simulink model "Mission_Server_QBot2e_IO_Check_r2018a"  (Simulink 9.1)
settings: Solver=ode2  StartTime=0.0  StopTime=inf  FixedStep=0.001  RelTol=1e-3  EnableMultiTasking=on
undefined symbols (not defined in the file): Host
libraries: quarc_library x13, simulink x4
settings Model: Creator=Admin  LastModifiedBy=user  SimulationMode=external  ExtModeTrigDuration=10000
settings SolverCC: PositivePriorityOrder=on
settings DataIOCC: SaveFormat=Dataset
settings OptimizationCC: LifeSpan=auto
settings DebuggingCC: UnderspecifiedInitializationDetection=Simplified  MergeDetectMultiDrivingBlocksExec=error
settings HardwareCC: ProdBitPerPointer=64  ProdBitPerSizeT=64  ProdBitPerPtrDiffT=64  ProdLargestAtomicFloat=Float  ProdIntDivRoundTo=Zero  ProdEndianess=LittleEndian  ProdWordSize=64  ProdHWDeviceType=Intel->x86-64 (Windows64)
settings ModelReferenceCC: PropagateSignalLabelsOutOfModel=on
settings RTWCC: Description=QUARC Win64 Target Using Toolchain  SystemTargetFile=quarc_win64.tlc  TemplateMakefile=quarc_default_tmf  Toolchain=QUARC win64 | nmake (64-bit Windows)  BuildConfiguration=Faster Runs
settings STFCustomTargetCC: ConcurrentExecutionCompliant=on  UseToolchainInfoCompliant=on  SystemTargetFile=quarc_win64.tlc
settings GRTTargetCC: ParMdlRefBuildCompliant=off  CompOptLevelCompliant=off  MatFileLogging=off  CPPClassGenCompliant=off  ExtMode=on  ExtModeMexFile=quarc_comm  ExtModeMexArgs='-w -d %d -uri %u -d_IP_q tcpip://localhost:18000'

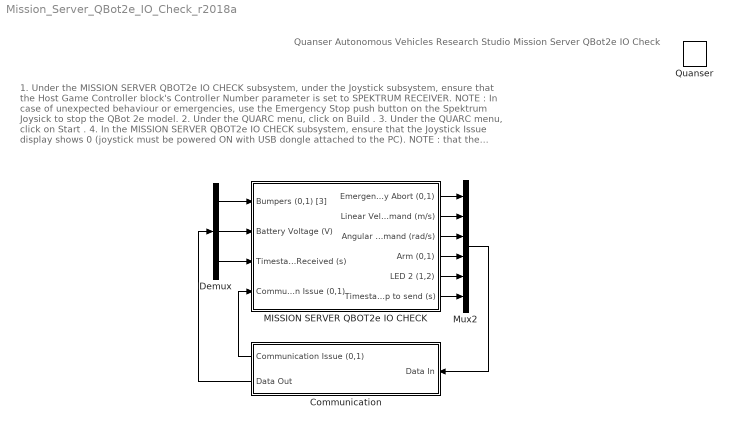
== system Mission_Server_QBot2e_IO_Check_r2018a ==
  note: 1. Under the MISSION SERVER QBOT2e IO CHECK subsystem, under the Joystick subsystem, ensure that the Host Game Controller block's Controller Number parameter is set to SPEKTRUM RECEIVER.
      | NOTE : In case of unexpected behaviour or emergencies, use the Emergency Stop push button on the Spektrum Joysick to stop the QBot 2e model.
      | 2. Under the QUARC menu, click on Build .
      | 3. Under the QUARC menu, click on Start .
      | 4. In the MISSION SERVER QBOT2e IO CHECK subsystem, ensure that the Joystick Issue display shows 0 (joystick must be powered ON with USB dongle attached to the PC).
      | NOTE : that the Loop-back Time (s) display SHOULD display an increasing time value until the QBot 2e Stabilizer model is running. When it is running, this display should oscillate around a small value (~0.004 to 0.005s).
  note: Quanser Autonomous Vehicles Research Studio
      | Mission Server QBot2e IO Check
  Communication : Subsystem
  Demux : Demux  Outputs=[3 1 1 ]
  MISSION SERVER QBOT2e IO CHECK : Subsystem
  Mux2 : Mux  Inputs=6
  Quanser : quarc_library/Logos/Quanser
  wires:
  Communication/2(Data Out) -> Demux/1
  Demux/3 -> MISSION SERVER QBOT2e IO CHECK/3(Timestamp Received (s))
  Demux/1 -> MISSION SERVER QBOT2e IO CHECK/1(Bumpers (0,1) [3])
  Demux/2 -> MISSION SERVER QBOT2e IO CHECK/2(Battery Voltage (V))
  Communication/1(Communication Issue (0,1)) -> MISSION SERVER QBOT2e IO CHECK/4(Communication Issue (0,1))
  MISSION SERVER QBOT2e IO CHECK/1(Emergency Abort (0,1)) -> Mux2/1
  MISSION SERVER QBOT2e IO CHECK/2(Linear Velocity Command (m/s)) -> Mux2/2
  MISSION SERVER QBOT2e IO CHECK/3(Angular Velocity Command (rad/s)) -> Mux2/3
  MISSION SERVER QBOT2e IO CHECK/4(Arm (0,1)) -> Mux2/4
  MISSION SERVER QBOT2e IO CHECK/5(LED 2 (1,2)) -> Mux2/5
  MISSION SERVER QBOT2e IO CHECK/6(Timestamp to send (s)) -> Mux2/6
  Mux2/1 -> Communication/1(Data In)

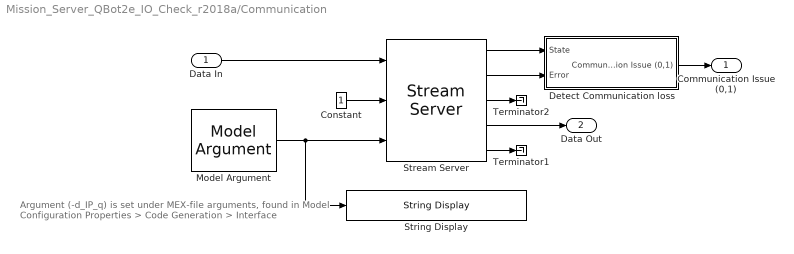
== system Mission_Server_QBot2e_IO_Check_r2018a/Communication ==
  note: Argument (-d_IP_q) is set under
      | MEX-file arguments, found in
      | Model Configuration Properties > Code Generation > Interface
  Data In : Inport
  Constant : Constant
  Detect Communication loss : Subsystem
  Model Argument : quarc_library/Sources/Signals/Model Argument  argument_name=d_IP_q  has_value=on  data_type_mode=Specify via dialog  data_type=char  max_length=80  default_value=0  variable_size=off
      settings: AttributesFormatString=(-%<argument_name>)  SourceProductName=QUARC Targets
  Stream Server : quarc_library/Communications/Basic/Stream Server  uri_source=External input port  uri=tcpip://localhost:18666  apply_uri_to_all_configs=off  send_buffer_size=1460  receive_buffer_size=1460  byte_order=little endian (Intel - LSB first)  optimization=Minimum latency  send_options=Send most recent data  receive_options=Receive most recent data  default_value=zeros(1,5)  sample_time=qc_get_step_size  active=off  implementation=Use blocking I/O in a separate thread  send_fifo_size=1  receive_fifo_size=1  send_priority=0  receive_priority=0  send_dimensions=off  receive_dimensions=off  max_dimensions=-1  data_type=double  type_expr=BusObject
  "String Display " : quarc_library/Strings/String Display  alignment=center  display_mode=Single line  sample_time=-1  use_new=off
      settings: SourceProductName=QUARC Targets
  Terminator1 : Terminator
  Terminator2 : Terminator
  Communication Issue (0,1) : Outport  VectorParamsAs1DForOutWhenUnconnected=off
  Data Out : Outport  Port=2  VectorParamsAs1DForOutWhenUnconnected=off
  wires:
  Stream Server/3 -> Terminator2/1
  Constant/1 -> Stream Server/2
  Stream Server/1 -> Detect Communication loss/1(State)
  Data In/1 -> Stream Server/1
  Model Argument/1 -> Stream Server/3, "String Display "/1
  Stream Server/4 -> Data Out/1
  Stream Server/5 -> Terminator1/1
  Stream Server/2 -> Detect Communication loss/2(Error)
  Detect Communication loss/1(Communication Issue (0,1)) -> Communication Issue (0,1)/1

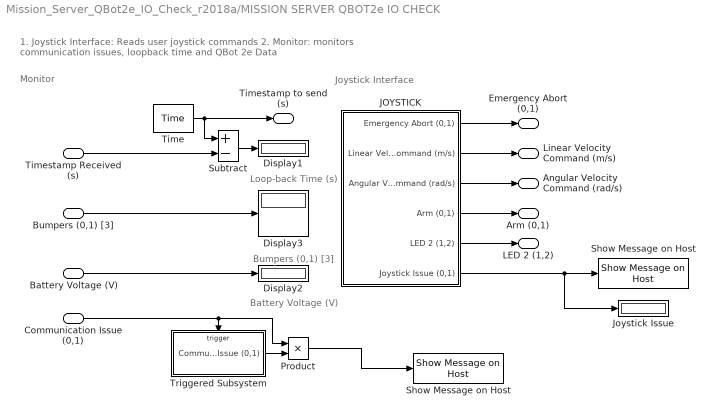
== system Mission_Server_QBot2e_IO_Check_r2018a/MISSION SERVER QBOT2e IO CHECK ==
  note: Monitor
  note: Joystick Interface
  note: 1. Joystick Interface: Reads user joystick commands
      | 2. Monitor: monitors communication issues, loopback time and QBot 2e Data
  note: Battery Voltage (V)
  note: Bumpers (0,1) [3]
  note: Loop-back Time (s)
  Bumpers (0,1) [3] : Inport
  Battery Voltage (V) : Inport  Port=2
  Timestamp Received (s) : Inport  Port=3
  Communication Issue (0,1) : Inport  Port=4
  Display1 : Display
  Display2 : Display
  Display3 : Display
  JOYSTICK : Subsystem
  Joystick Issue : Display
  Product : Product
  Show Message on Host : quarc_library/Sinks/Error Handling/Show Message on Host  message_type=Fixed error message  message_icon=Warning  message=Mission Server: Communication Issue with QBot2e
      settings: AttributesFormatString="\"%<message>\""  SourceProductName=QUARC Targets
  "Show Message on Host " : quarc_library/Sinks/Error Handling/Show Message on Host  message_type=Fixed error message  message_icon=Warning  message=Mission Server: Joystick Disconnected
      settings: AttributesFormatString="\"%<message>\""  SourceProductName=QUARC Targets
  Subtract : Sum  Inputs=+-
  Time : quarc_library/Sources/Time/Time  time_source=Wall clock  sample_time=qc_get_step_size
  Triggered Subsystem : Subsystem  TreatAsAtomicUnit=on
  Emergency Abort (0,1) : Outport  VectorParamsAs1DForOutWhenUnconnected=off
  Linear Velocity Command (m/s) : Outport  Port=2  VectorParamsAs1DForOutWhenUnconnected=off
  Angular Velocity Command (rad/s) : Outport  Port=3  VectorParamsAs1DForOutWhenUnconnected=off
  Arm (0,1) : Outport  Port=4  VectorParamsAs1DForOutWhenUnconnected=off
  LED 2 (1,2) : Outport  Port=5  VectorParamsAs1DForOutWhenUnconnected=off
  Timestamp to send (s) : Outport  Port=6  VectorParamsAs1DForOutWhenUnconnected=off
  wires:
  JOYSTICK/6(Joystick Issue (0,1)) -> "Show Message on Host "/1, Joystick Issue/1
  Battery Voltage (V)/1 -> Display2/1
  Bumpers (0,1) [3]/1 -> Display3/1
  Communication Issue (0,1)/1 -> Product/1, Triggered Subsystem/Trigger
  Triggered Subsystem/1(Communication Issue (0,1)) -> Product/2
  Product/1 -> Show Message on Host/1
  Time/1 -> Timestamp to send (s)/1, Subtract/1
  Timestamp Received (s)/1 -> Subtract/2
  Subtract/1 -> Display1/1
  JOYSTICK/2(Linear Velocity Command (m/s)) -> Linear Velocity Command (m/s)/1
  JOYSTICK/1(Emergency Abort (0,1)) -> Emergency Abort (0,1)/1
  JOYSTICK/4(Arm (0,1)) -> Arm (0,1)/1
  JOYSTICK/3(Angular Velocity Command (rad/s)) -> Angular Velocity Command (rad/s)/1
  JOYSTICK/5(LED 2 (1,2)) -> LED 2 (1,2)/1

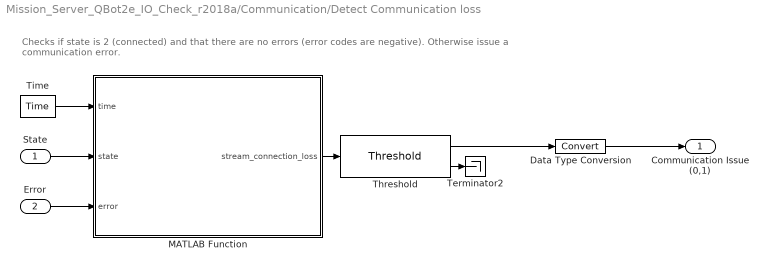
== system Mission_Server_QBot2e_IO_Check_r2018a/Communication/Detect Communication loss ==
  note: Checks if state is 2 (connected) and that there are no errors (error codes are negative). Otherwise issue a communication error.
  State : Inport
  Error : Inport  Port=2
  Data Type Conversion : DataTypeConversion
  MATLAB Function : MATLAB Function  TreatAsAtomicUnit=on
  Terminator2 : Terminator
  Threshold : quarc_library/Discontinuities/Threshold  operator=>=  param_src=Specify via dialog  threshold=0.5  duration=0.1
      settings: SourceProductName=QUARC Targets
  Time : quarc_library/Sources/Time/Time  time_source=Wall clock  sample_time=qc_get_step_size
  Communication Issue (0,1) : Outport  VectorParamsAs1DForOutWhenUnconnected=off
  wires:
  Error/1 -> MATLAB Function/3(error)
  MATLAB Function/1(stream_connection_loss) -> Threshold/1
  State/1 -> MATLAB Function/2(state)
  Time/1 -> MATLAB Function/1(time)
  Threshold/2 -> Terminator2/1
  Data Type Conversion/1 -> Communication Issue (0,1)/1
  Threshold/1 -> Data Type Conversion/1

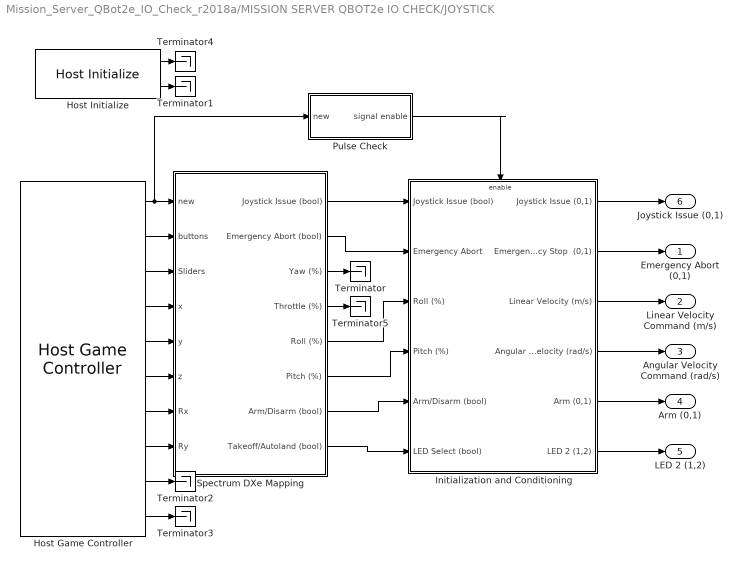
== system Mission_Server_QBot2e_IO_Check_r2018a/MISSION SERVER QBOT2e IO CHECK/JOYSTICK ==
  Host Game Controller : quarc_library/Devices/Peripherals/Host/Host Game Controller  object_name=Host-1  controller=1  buffer_size=20  deadzone=[]  saturation=[]  sample_time=qc_get_step_size  auto_center=off  enabled=on  debug_mode=off
      settings: SourceProductName=QUARC Targets
  Host Initialize : quarc_library/Devices/Peripherals/Host/Host Initialize  object_name=Host-1  uri_source=Use external mode communications  uri=tcpip://localhost:18001  apply_uri_to_all_configs=on  send_buffer_size=1000  receive_buffer_size=1000  thread_priority=0  run_client=on  use_window=off  window_position=[]  sample_time=qc_get_step_size  active=on
      settings: SourceProductName=QUARC Targets
  Initialization and Conditioning : Subsystem  TreatAsAtomicUnit=on
  Pulse Check : Subsystem
  Spectrum DXe Mapping : Subsystem
  Terminator{,1..5} (6 alike) : Terminator
  Emergency Abort (0,1) : Outport  VectorParamsAs1DForOutWhenUnconnected=off
  Linear Velocity Command (m/s) : Outport  Port=2  VectorParamsAs1DForOutWhenUnconnected=off
  Angular Velocity Command (rad/s) : Outport  Port=3  VectorParamsAs1DForOutWhenUnconnected=off
  Arm (0,1) : Outport  Port=4  VectorParamsAs1DForOutWhenUnconnected=off
  LED 2 (1,2) : Outport  Port=5  VectorParamsAs1DForOutWhenUnconnected=off
  Joystick Issue (0,1) : Outport  Port=6  VectorParamsAs1DForOutWhenUnconnected=off
  wires:
  Initialization and Conditioning/1(Joystick Issue (0,1)) -> Joystick Issue (0,1)/1
  Spectrum DXe Mapping/1(Joystick Issue (bool)) -> Initialization and Conditioning/1(Joystick Issue (bool))
  Host Game Controller/7 -> Spectrum DXe Mapping/7(Rx)
  Host Game Controller/10 -> Terminator3/1
  Host Game Controller/9 -> Terminator2/1
  Host Game Controller/8 -> Spectrum DXe Mapping/8(Ry)
  Host Game Controller/4 -> Spectrum DXe Mapping/4(x)
  Host Game Controller/5 -> Spectrum DXe Mapping/5(y)
  Host Game Controller/3 -> Spectrum DXe Mapping/3(Sliders)
  Host Game Controller/6 -> Spectrum DXe Mapping/6(z)
  Host Initialize/1 -> Terminator4/1
  Host Initialize/2 -> Terminator1/1
  Spectrum DXe Mapping/7("Arm/Disarm (bool) ") -> Initialization and Conditioning/5(Arm/Disarm (bool))
  Spectrum DXe Mapping/5(Roll (%)) -> Initialization and Conditioning/3(Roll (%))
  Spectrum DXe Mapping/6(Pitch (%)) -> Initialization and Conditioning/4(Pitch (%))
  Host Game Controller/2 -> Spectrum DXe Mapping/2(buttons)
  Spectrum DXe Mapping/2(Emergency Abort (bool)) -> Initialization and Conditioning/2(Emergency Abort)
  Spectrum DXe Mapping/8(Takeoff/Autoland (bool)) -> Initialization and Conditioning/6(LED Select (bool))
  Initialization and Conditioning/2("Emergency Stop  (0,1) ") -> Emergency Abort (0,1)/1
  Initialization and Conditioning/3(Linear Velocity (m/s)) -> Linear Velocity Command (m/s)/1
  Initialization and Conditioning/5("Arm (0,1) ") -> Arm (0,1)/1
  Initialization and Conditioning/6(LED 2 (1,2)) -> LED 2 (1,2)/1
  Initialization and Conditioning/4(Angular Velocity (rad/s)) -> Angular Velocity Command (rad/s)/1
  Spectrum DXe Mapping/3(Yaw (%)) -> Terminator/1
  Spectrum DXe Mapping/4(Throttle (%)) -> Terminator5/1
  Pulse Check/1("signal enable ") -> Initialization and Conditioning/Enable
  Host Game Controller/1 -> Pulse Check/1(new), Spectrum DXe Mapping/1(new)

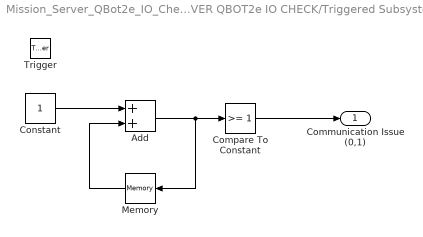
== system Mission_Server_QBot2e_IO_Check_r2018a/MISSION SERVER QBOT2e IO CHECK/Triggered Subsystem ==
  Trigger : TriggerPort  TriggerType=falling  VariantControl=Variant
  Add : Sum
  Compare To Constant : simulink/Logic and Bit Operations/Compare To Constant  relop=>=  const=1  OutDataTypeStr=boolean
  Constant : Constant
  Memory : Memory  InheritSampleTime=on
  Communication Issue (0,1) : Outport  InitialOutput=0  VectorParamsAs1DForOutWhenUnconnected=off
  wires:
  Constant/1 -> Add/1
  Memory/1 -> Add/2
  Add/1 -> Compare To Constant/1, Memory/1
  Compare To Constant/1 -> Communication Issue (0,1)/1

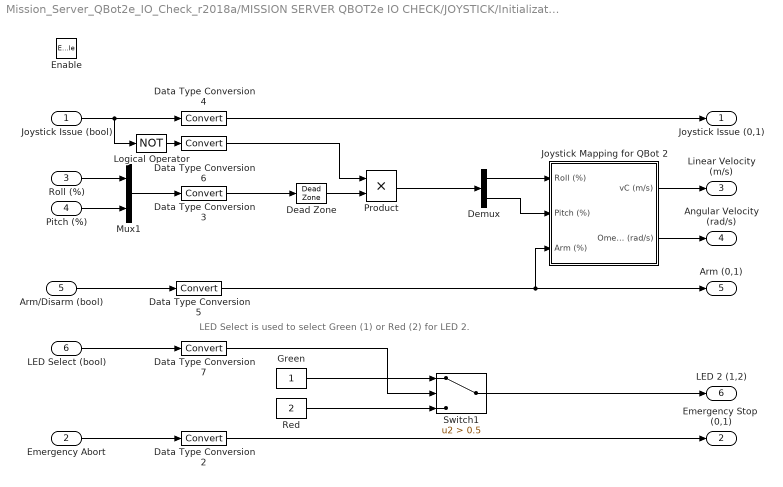
== system Mission_Server_QBot2e_IO_Check_r2018a/MISSION SERVER QBOT2e IO CHECK/JOYSTICK/Initialization and Conditioning ==
  note: LED Select is used to select Green (1) or Red (2) for LED 2.
  Joystick Issue (bool) : Inport
  Emergency Abort : Inport  Port=2
  Roll (%) : Inport  Port=3
  Pitch (%) : Inport  Port=4
  Arm/Disarm (bool) : Inport  Port=5
  LED Select (bool) : Inport  Port=6
  Enable : EnablePort  StatesWhenEnabling=reset
  Data Type Conversion{2..7} (6 alike) : DataTypeConversion
  Dead Zone : DeadZone  LowerValue=-0.01  UpperValue=0.01  SaturateOnIntegerOverflow=on
  Demux : Demux  Outputs=2
  Green : Constant
  Joystick Mapping for QBot 2 : Subsystem
  Logical Operator : Logic  Operator=NOT  AllPortsSameDT=off  OutDataTypeStr=boolean
  Mux1 : Mux  Inputs=2
  Product : Product
  Red : Constant  Value=2
  Switch1 : Switch  Criteria=u2 > Threshold  Threshold=0.5
  Joystick Issue (0,1) : Outport  InitialOutput=0  VectorParamsAs1DForOutWhenUnconnected=off
  "Emergency Stop  (0,1) " : Outport  Port=2  InitialOutput=0  VectorParamsAs1DForOutWhenUnconnected=off
  Linear Velocity (m/s) : Outport  Port=3  InitialOutput=0  VectorParamsAs1DForOutWhenUnconnected=off
  Angular Velocity (rad/s) : Outport  Port=4  InitialOutput=0  VectorParamsAs1DForOutWhenUnconnected=off
  "Arm (0,1) " : Outport  Port=5  InitialOutput=0  VectorParamsAs1DForOutWhenUnconnected=off
  LED 2 (1,2) : Outport  Port=6  InitialOutput=0  VectorParamsAs1DForOutWhenUnconnected=off
  wires:
  Joystick Issue (bool)/1 -> Data Type Conversion4/1, Logical Operator/1
  Mux1/1 -> Data Type Conversion3/1
  Roll (%)/1 -> Mux1/1
  Pitch (%)/1 -> Mux1/2
  Data Type Conversion4/1 -> Joystick Issue (0,1)/1
  Emergency Abort/1 -> Data Type Conversion2/1
  Data Type Conversion3/1 -> Dead Zone/1
  Arm/Disarm (bool)/1 -> Data Type Conversion5/1
  Logical Operator/1 -> Data Type Conversion6/1
  Dead Zone/1 -> Product/2
  Data Type Conversion6/1 -> Product/1
  Data Type Conversion5/1 -> Joystick Mapping for QBot 2/3(Arm (%)), "Arm (0,1) "/1
  LED Select (bool)/1 -> Data Type Conversion7/1
  Demux/1 -> Joystick Mapping for QBot 2/1(Roll (%))
  Demux/2 -> Joystick Mapping for QBot 2/2(Pitch (%))
  Product/1 -> Demux/1
  Data Type Conversion7/1 -> Switch1/2
  Data Type Conversion2/1 -> "Emergency Stop  (0,1) "/1
  Joystick Mapping for QBot 2/1(vC (m/s)) -> Linear Velocity (m/s)/1
  Joystick Mapping for QBot 2/2(Omega (rad/s)) -> Angular Velocity (rad/s)/1
  Switch1/1 -> LED 2 (1,2)/1
  Green/1 -> Switch1/1
  Red/1 -> Switch1/3

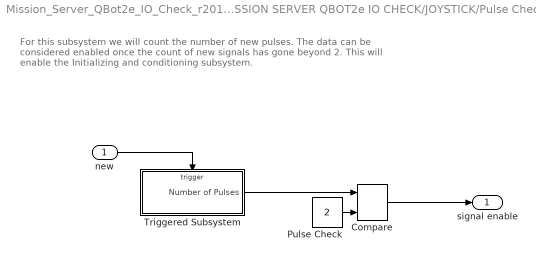
== system Mission_Server_QBot2e_IO_Check_r2018a/MISSION SERVER QBOT2e IO CHECK/JOYSTICK/Pulse Check ==
  note: For this subsystem we will count the number of new pulses. The data can be considered enabled once the count of new signals has gone beyond 2. This will enable the Initializing and conditioning subsystem.
  new : Inport
  Compare : quarc_library/Logic Operations/Compare  operator=>  output_data_type=boolean
      settings: SourceProductName=QUARC Targets
  "Pulse Check  " : Constant  Value=2
  Triggered Subsystem : Subsystem  TreatAsAtomicUnit=on
  "signal enable " : Outport  VectorParamsAs1DForOutWhenUnconnected=off
  wires:
  "Pulse Check  "/1 -> Compare/2
  Compare/1 -> "signal enable "/1
  Triggered Subsystem/1(Number of Pulses) -> Compare/1
  new/1 -> Triggered Subsystem/Trigger

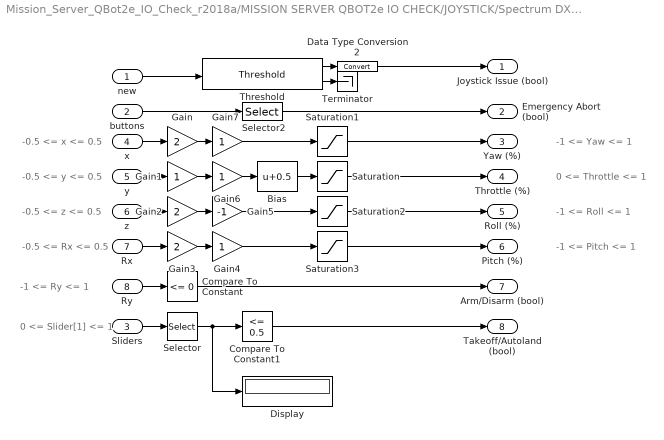
== system Mission_Server_QBot2e_IO_Check_r2018a/MISSION SERVER QBOT2e IO CHECK/JOYSTICK/Spectrum DXe Mapping ==
  note: -0.5 <= x <= 0.5
  note: -1 <= Yaw <= 1
  note: -0.5 <= y <= 0.5
  note: 0 <= Throttle <= 1
  note: -0.5 <= z <= 0.5
  note: -1 <= Roll <= 1
  note: -0.5 <= Rx <= 0.5
  note: -1 <= Pitch <= 1
  note: 0 <= Slider[1] <= 1
  note: -1 <= Ry <= 1
  new : Inport
  buttons : Inport  Port=2
  Sliders : Inport  Port=3
  x : Inport  Port=4
  y : Inport  Port=5
  z : Inport  Port=6
  Rx : Inport  Port=7
  Ry : Inport  Port=8
  Bias : Bias  Bias=0.5
  Compare To Constant : simulink/Logic and Bit Operations/Compare To Constant  relop=<=  const=0  OutDataTypeStr=boolean
  Compare To Constant1 : simulink/Logic and Bit Operations/Compare To Constant  relop=<=  const=0.5  OutDataTypeStr=boolean
  Data Type Conversion2 : DataTypeConversion
  Display : Display
  Gain : Gain  Gain=2
  Gain{1,4,6..7} (4 alike) : Gain
  Gain2 : Gain  Gain=2
  Gain3 : Gain  Gain=2
  Gain5 : Gain  Gain=-1
  Saturation : Saturate  UpperLimit=1  LowerLimit=0
  Saturation1 : Saturate  UpperLimit=1  LowerLimit=-1
  Saturation2 : Saturate  UpperLimit=1  LowerLimit=-1
  Saturation3 : Saturate  UpperLimit=1  LowerLimit=-1
  Selector : Selector  InputPortWidth=2  IndexOptions=Index vector (dialog)  Indices=[1]  OutputSizes=1
  Selector2 : Selector  InputPortWidth=32  IndexOptions=Index vector (dialog)  Indices=[1]  OutputSizes=1
  Terminator : Terminator
  Threshold : quarc_library/Discontinuities/Threshold  operator===  param_src=Specify via dialog  threshold=0  duration=1
      settings: SourceProductName=QUARC Targets
  Joystick Issue (bool) : Outport  VectorParamsAs1DForOutWhenUnconnected=off
  Emergency Abort (bool) : Outport  Port=2  VectorParamsAs1DForOutWhenUnconnected=off
  Yaw (%) : Outport  Port=3  VectorParamsAs1DForOutWhenUnconnected=off
  Throttle (%) : Outport  Port=4  VectorParamsAs1DForOutWhenUnconnected=off
  Roll (%) : Outport  Port=5  VectorParamsAs1DForOutWhenUnconnected=off
  Pitch (%) : Outport  Port=6  VectorParamsAs1DForOutWhenUnconnected=off
  "Arm/Disarm (bool) " : Outport  Port=7  VectorParamsAs1DForOutWhenUnconnected=off
  Takeoff/Autoland (bool) : Outport  Port=8  VectorParamsAs1DForOutWhenUnconnected=off
  wires:
  Compare To Constant/1 -> "Arm/Disarm (bool) "/1
  Saturation3/1 -> Pitch (%)/1
  Gain7/1 -> Saturation1/1
  Selector/1 -> Display/1, Compare To Constant1/1
  Gain5/1 -> Saturation2/1
  Saturation/1 -> Throttle (%)/1
  Sliders/1 -> Selector/1
  Gain6/1 -> Bias/1
  Saturation1/1 -> Yaw (%)/1
  Gain/1 -> Gain7/1
  Gain3/1 -> Gain4/1
  Saturation2/1 -> Roll (%)/1
  Bias/1 -> Saturation/1
  Gain2/1 -> Gain5/1
  Gain1/1 -> Gain6/1
  Gain4/1 -> Saturation3/1
  z/1 -> Gain2/1
  x/1 -> Gain/1
  Ry/1 -> Compare To Constant/1
  y/1 -> Gain1/1
  Rx/1 -> Gain3/1
  Compare To Constant1/1 -> Takeoff/Autoland (bool)/1
  buttons/1 -> Selector2/1
  Threshold/2 -> Terminator/1
  Selector2/1 -> Emergency Abort (bool)/1
  Threshold/1 -> Data Type Conversion2/1
  new/1 -> Threshold/1
  Data Type Conversion2/1 -> Joystick Issue (bool)/1

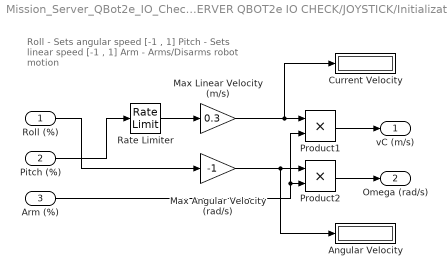
== system Mission_Server_QBot2e_IO_Check_r2018a/MISSION SERVER QBOT2e IO CHECK/JOYSTICK/Initialization and Conditioning/Joystick Mapping for QBot 2 ==
  note: Roll		- Sets angular speed  	[-1		, 1]
      | Pitch	- Sets linear speed  	[-1		, 1]
      | Arm		- Arms/Disarms robot motion
  Roll (%) : Inport
  Pitch (%) : Inport  Port=2
  Arm (%) : Inport  Port=3
  Angular Velocity : Display
  Current Velocity : Display
  Max Angular Velocity (rad/s) : Gain  Gain=-1
  Max Linear Velocity (m/s) : Gain  Gain=0.3
  Product1 : Product
  Product2 : Product
  Rate Limiter : RateLimiter  RisingSlewLimit=2  FallingSlewLimit=-2  SampleTimeMode=inherited
  vC (m/s) : Outport  VectorParamsAs1DForOutWhenUnconnected=off
  Omega (rad/s) : Outport  Port=2  VectorParamsAs1DForOutWhenUnconnected=off
  wires:
  Product2/1 -> Omega (rad/s)/1
  Roll (%)/1 -> Max Angular Velocity (rad/s)/1
  Pitch (%)/1 -> Rate Limiter/1
  Max Linear Velocity (m/s)/1 -> Current Velocity/1, Product1/1
  Max Angular Velocity (rad/s)/1 -> Angular Velocity/1, Product2/1
  Arm (%)/1 -> Product1/2, Product2/2
  Rate Limiter/1 -> Max Linear Velocity (m/s)/1
  Product1/1 -> vC (m/s)/1

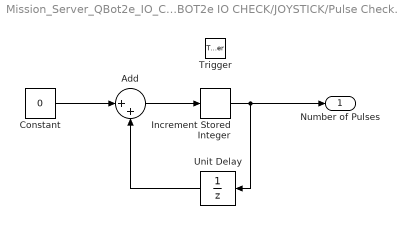
== system Mission_Server_QBot2e_IO_Check_r2018a/MISSION SERVER QBOT2e IO CHECK/JOYSTICK/Pulse Check/Triggered Subsystem ==
  Trigger : TriggerPort  VariantControl=Variant
  Add : Sum  Inputs=|++
  Constant : Constant  Value=0
  Increment Stored Integer : simulink/Additional Math & Discrete/Additional Math: Increment - Decrement/Increment Stored Integer
  Unit Delay : UnitDelay  SampleTime=-1  HasFrameUpgradeWarning=on
  Number of Pulses : Outport  VectorParamsAs1DForOutWhenUnconnected=off
  wires:
  Unit Delay/1 -> Add/2
  Increment Stored Integer/1 -> Unit Delay/1, Number of Pulses/1
  Add/1 -> Increment Stored Integer/1
  Constant/1 -> Add/1

== matlab function Communication/Detect Communication loss/MATLAB Function ==
  data: time input double; stream_connection_loss output double; state input double; error input double
function stream_connection_loss  = fcn(time, state, error)

stream_connection_loss = 0;
if time > 1
    if ~((state == 2)&&(error >= 0))
        % stream connection is not established correctly
        stream_connection_loss = 1;
    end
end
